simulink model "speed_control_of_dc_motor"  (R2018b)
settings: Solver=FixedStepDiscrete  StartTime=0.0  StopTime=inf  FixedStep=0.0005  RelTol=1e-3  EnableMultiTasking=on
libraries: arduinolib x5, simulink x2
settings Model: ExtModeTrigDuration=2  Creator=avata  LastModifiedBy=Atef
settings DataIOCC: ReturnWorkspaceOutputs=on
settings OptimizationCC: EnhancedBackFolding=on  PassReuseOutputArgsAs=Individual arguments  ZeroExternalMemoryAtStartup=off  ZeroInternalMemoryAtStartup=off  MaxStackSize=64  OptimizeBlockOrder=speed  DifferentSizesBufferReuse=on  OptimizationCustomize=off
settings DebuggingCC: ParameterOverflowMsg=none  ParameterTunabilityLossMsg=error  SFMachineParentedDataDiag=error
settings HardwareCC: ProdBitPerInt=16  ProdBitPerPointer=16  ProdBitPerSizeT=16  ProdBitPerPtrDiffT=16  ProdLargestAtomicFloat=None  ProdWordSize=8  ProdHWDeviceType=Atmel->AVR
settings SFSimCC: MATLABDynamicMemAlloc=off
settings RTWCC: SystemTargetFile=ert.tlc  HardwareBoard=Arduino Uno  TemplateMakefile=ert_default_tmf  Toolchain=Arduino AVR  BuildConfiguration=Faster Runs
settings CodeAppCC: ForceParamTrailComments=on  IgnoreCustomStorageClasses=off  OperatorAnnotations=on  SimulinkDataObjDesc=on  SFDataObjDesc=on  InsertBlockDesc=on
settings ERTTargetCC: SupportContinuousTime=on  SupportVariableSizeSignals=on  ExtModeStaticAllocSize=250

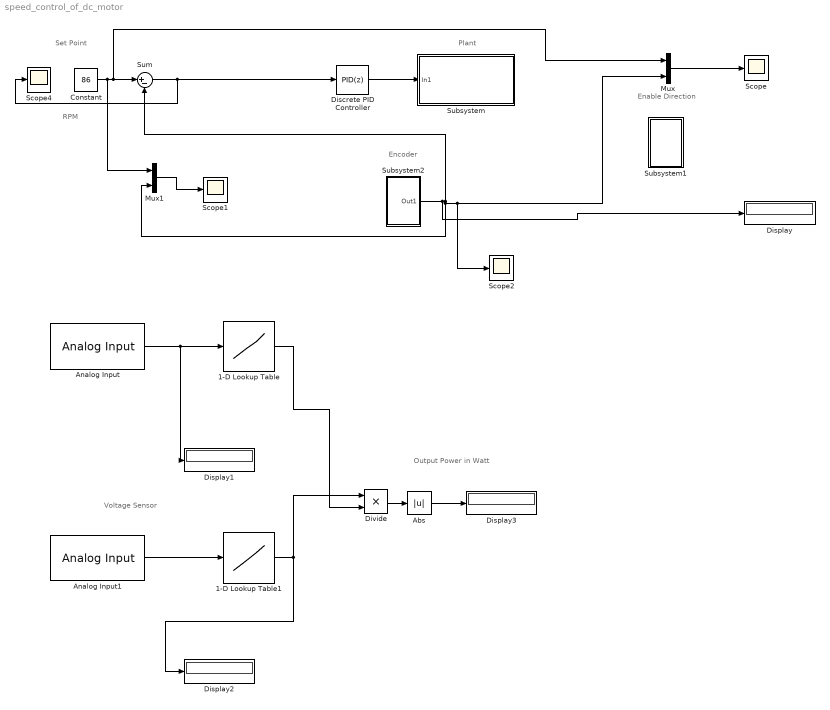
== system speed_control_of_dc_motor ==
  note: RPM
  note: Plant
  note: Set Point
  note: Encoder
  note: Enable Direction
  note: Output Power in Watt
  note: Voltage Sensor
  1-D Lookup Table : Lookup_n-D  NumberOfTableDimensions=1  BreakpointsForDimension1=[0,1.136666666666667e+02,2.273333333333333e+02,341,4.546666666666667e+02,5.683333333333334e+02,682,7.956666666666666e+02,9.093333333333334e+02,1023]  BreakpointsForDimension1FirstPoint=-5  BreakpointsForDimension1Spacing=1/102  Table=[-5,-3.888888888888889,-2.777777777777778,-1.666666666666667,-0.555555555555556,0.555555555555556,1.666666666666667,2.777777777777778,3.888888888888889,5]  ExtrapMethod=Clip  InternalRulePriority=Speed  RndMeth=Simplest  InputSameDT=on
  1-D Lookup Table1 : Lookup_n-D  NumberOfTableDimensions=1  BreakpointsForDimension1=[0,1.136666666666667e+02,2.273333333333333e+02,341,4.546666666666667e+02,5.683333333333334e+02,682,7.956666666666666e+02,9.093333333333334e+02,1023]  BreakpointsForDimension1FirstPoint=-5  BreakpointsForDimension1Spacing=1/102  Table=[0,2.777777777777778,5.555555555555555,8.333333333333334,11.111111111111110,13.888888888888890,16.666666666666668,19.444444444444443,22.222222222222220,25]  ExtrapMethod=Clip  InternalRulePriority=Speed  RndMeth=Simplest  InputSameDT=on
  Abs : Abs
  Analog Input : arduinolib/Analog Input  pinNumber=5  ReadResultsOnly=off  ConversionTriggerSource=Software  ExternalTriggerType=uint32( 0 )  OutputDataType=uint16  EnableConversionCompleteNotify=off  EnableOuputStatus=off  SampleTime=-1  blockPlatform=arduino
  Analog Input1 : arduinolib/Analog Input  pinNumber=4  ReadResultsOnly=off  ConversionTriggerSource=Software  ExternalTriggerType=uint32( 0 )  OutputDataType=uint16  EnableConversionCompleteNotify=off  EnableOuputStatus=off  SampleTime=-1  blockPlatform=arduino
  Constant : Constant  Value=86
  Discrete PID Controller : simulink/Continuous/PID Controller  Controller=PID  Form=Parallel  TimeDomain=Discrete-time  SampleTime=-1  IntegratorMethod=Forward Euler  FilterMethod=Forward Euler  ControllerParametersSource=internal  P=5  I=3  D=0  UseFilter=on  N=100  TunerSelectOption=Transfer Function Based (PID Tuner App)  InitialConditionSource=internal  InitialConditionForIntegrator=0  InitialConditionForFilter=0  DifferentiatorICPrevScaledInput=0  ExternalReset=none  TrackingMode=off  Kt=1  LimitOutput=off  UpperSaturationLimit=inf  LowerSaturationLimit=-inf  LinearizeAsGain=off  AntiWindupMode=none  Kb=1  POutMin=[]  POutMax=[]  IOutMin=[]  IOutMax=[]  DOutMin=[]  DOutMax=[]  NOutMin=[]  NOutMax=[]  SumOutMin=[]  SumOutMax=[]  SaturationOutMin=[]  SaturationOutMax=[]  PParamMin=[]  PParamMax=[]  IParamMin=[]  IParamMax=[]  DParamMin=[]  DParamMax=[]  NParamMin=[]  NParamMax=[]  KbParamMin=[]  KbParamMax=[]  KtParamMin=[]  KtParamMax=[]  KbOutMin=[]  KbOutMax=[]  KtOutMin=[]  KtOutMax=[]  IntegratorOutMin=[]  IntegratorOutMax=[]  FilterOutMin=[]  FilterOutMax=[]  SumI1OutMin=[]  SumI1OutMax=[]  SumI2OutMin=[]  SumI2OutMax=[]  SumI3OutMin=[]  SumI3OutMax=[]  SumI4OutMin=[]  SumI4OutMax=[]  SumDOutMin=[]  SumDOutMax=[]  DifferentiatorOutMin=[]  DifferentiatorOutMax=[]  FilterDiffOutCoefMin=[]  FilterDiffOutCoefMax=[]  ReciprocalOutMin=[]  ReciprocalOutMax=[]  SumDenOutMin=[]  SumDenOutMax=[]  SumNumOutMin=[]  SumNumOutMax=[]  DivideOutMin=[]  DivideOutMax=[]  IntegratorContinuousStateAttributes=''  IntegratorStateMustResolveToSignalObject=off  IntegratorRTWStateStorageClass=Auto  FilterContinuousStateAttributes=''  FilterStateMustResolveToSignalObject=off  FilterRTWStateStorageClass=Auto  ParallelPVariant=InternalParameters  IdealPVariant=Disabled  IVariant=InternalParameters  DVariant=InternalParameters  IntegratorVariant=Discrete  SatVariant=Disabled  AWVariant=Passthrough  PCopyVariant=Disabled  TRVariant=Disabled  FdbkBlocksVariant=Forward  IdealPFdbkVariant=Disabled  SatFdbkVariant=Disabled  DerivativeFilterVariant=ForwardEulerFilter  NVariant=InternalParameters  NCopyVariant=Disabled  FilterICVariant=InternalICsFilter  IntegratorICVariant=InternalICs  ExternalResetVariant=Disabled  TRSumVariant=Passthrough  SumFdbkVariant=Disabled  SumVariant=Sum_PID
  Display{,1..3} (4 alike) : Display
  Divide : Product  Inputs=**
  Mux : Mux  Inputs=2
  Mux1 : Mux  Inputs=2
  Scope{,1..2,4} (4 alike) : Scope
  Subsystem : Subsystem
  Subsystem1 : Subsystem
  Subsystem2 : Subsystem
  Sum : Sum  Inputs=|+-
  wires:
  Sum/1 -> Scope4/1, Discrete PID Controller/1
  Mux/1 -> Scope/1
  Discrete PID Controller/1 -> Subsystem/1(In1)
  1-D Lookup Table/1 -> Divide/2
  Analog Input1/1 -> 1-D Lookup Table1/1
  1-D Lookup Table1/1 -> Divide/1, Display2/1
  Divide/1 -> Abs/1
  Abs/1 -> Display3/1
  Constant/1 -> Mux1/1, Mux/1, Sum/1
  Subsystem2/1(Out1) -> Display/1, Mux1/2, Scope2/1, Mux/2, Sum/2
  Mux1/1 -> Scope1/1
  Analog Input/1 -> Display1/1, 1-D Lookup Table/1

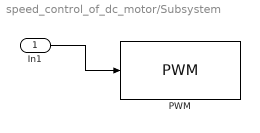
== system speed_control_of_dc_motor/Subsystem ==
  In1 : Inport
  PWM : arduinolib/PWM  pinNumber=5  EnableInputFrequency=off  InitialFrequency=2000  InitialDutyCycle=0  NotificationType=None  blockPlatform=arduino
  wires:
  In1/1 -> PWM/1

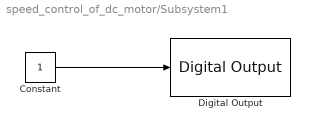
== system speed_control_of_dc_motor/Subsystem1 ==
  Constant : Constant
  Digital Output : arduinolib/Digital Output  pinNumber=9  blockPlatform=arduino
  wires:
  Constant/1 -> Digital Output/1

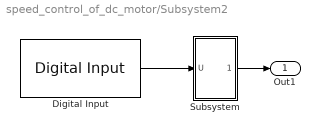
== system speed_control_of_dc_motor/Subsystem2 ==
  Digital Input : arduinolib/Digital Input  pinNumber=2  sampleTime=-1  blockPlatform=arduino
  Subsystem : Subsystem
  Out1 : Outport  VectorParamsAs1DForOutWhenUnconnected=on
  wires:
  Subsystem/1(Out1) -> Out1/1
  Digital Input/1 -> Subsystem/1(U)

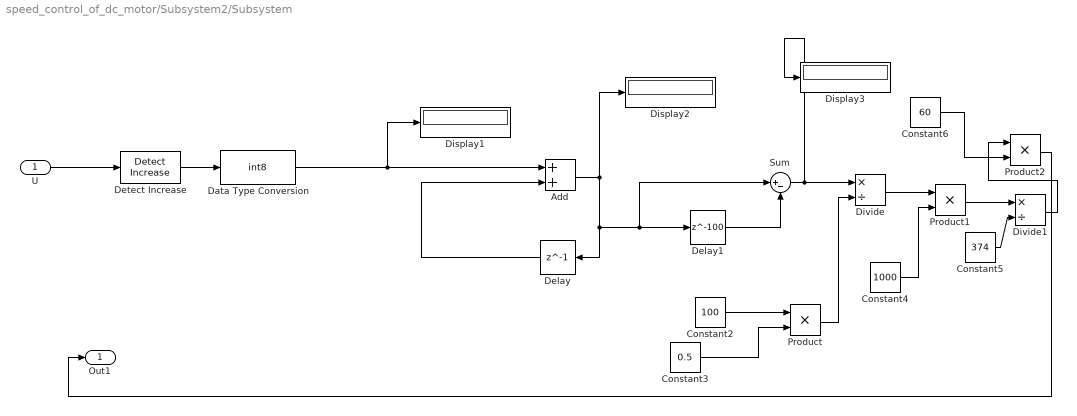
== system speed_control_of_dc_motor/Subsystem2/Subsystem ==
  U : Inport
  Add : Sum
  Constant2 : Constant  Value=100
  Constant3 : Constant  Value=0.5
  Constant4 : Constant  Value=1000
  Constant5 : Constant  Value=374
  Constant6 : Constant  Value=60
  Data Type Conversion : DataTypeConversion  OutDataTypeStr=int8
  Delay : Delay  DelayLength=1
  Delay1 : Delay  DelayLength=100
  Detect Increase : simulink/Logic and Bit Operations/Detect Increase  vinit=0.0  OutDataTypeStr=boolean
  Display1 : Display
  Display2 : Display
  Display3 : Display
  Divide : Product  Inputs=*/
  Divide1 : Product  Inputs=*/
  Product : Product
  Product1 : Product
  Product2 : Product
  Sum : Sum  Inputs=|+-
  Out1 : Outport  VectorParamsAs1DForOutWhenUnconnected=on
  wires:
  Divide1/1 -> Product2/1
  Data Type Conversion/1 -> Display1/1, Add/1
  Constant6/1 -> Product2/2
  Product/1 -> Divide/2
  Product1/1 -> Divide1/1
  Sum/1 -> Display3/1, Divide/1
  Add/1 -> Display2/1, Sum/1, Delay1/1, Delay/1
  Constant3/1 -> Product/2
  Delay1/1 -> Sum/2
  Detect Increase/1 -> Data Type Conversion/1
  Constant2/1 -> Product/1
  Divide/1 -> Product1/1
  Constant4/1 -> Product1/2
  Constant5/1 -> Divide1/2
  Product2/1 -> Out1/1
  Delay/1 -> Add/2
  U/1 -> Detect Increase/1
